simulink model "RTex"  (Simulink 6.0)
settings: Solver=ode3  StartTime=0.0  StopTime=10  FixedStep=0.25  RelTol=1e-3
settings Model: LastModifiedBy=ugur  ExtModeTrigMode=oneshot  ExtModeArmWhenConnect=off
settings ConfigSet: SimulationMode=accelerator
settings DataIOCC: LimitDataPoints=off  SignalLoggingName=sigsOut
settings OptimizationCC: BlockReduction=off  BooleanDataType=off  InlineInvariantSignals=off  LocalBlockOutputs=off
settings DebuggingCC: SolverPrmCheckMsg=none
settings HardwareCC: TargetHWDeviceType=32-bit Generic  ProdEqTarget=off
settings RTWCC: MakeCommand="make_rtw S_FUNCTIONS_LIB=\"..\\rt.lib ..\\winmm.lib\""

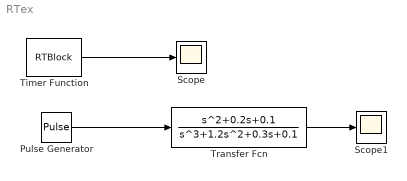
== system RTex ==
  Pulse Generator : DiscretePulseGenerator  PulseType=Time based  Period=1  PulseWidth=50
  Scope : Scope
      settings: YMin=0  YMax=500  SaveName=timing  DataFormat=Array
  Scope1 : Scope
      settings: YMin=0.375  YMax=0.625
  Timer Function : S-Function  FunctionName=RTBlock  Parameters=step,priority,ThPriority  mask(RTBlock){step=250, priority=NORMAL, ThPriority=NORMAL}
      mask prompts: step "Timestep (ms)"; ThPriority "Thread Priority"
      mask help:
      | Real Time Block: Set the characteristics of a real-time simulation. The settings of the simulation are selectable using the block panel. The parameters are:
      |
      | - Timeout: in milliseconds, defines the temporization with which Simulink requires to the Operating System the availability of resources for the execution of the simulation step. The value should be fixed equal to the simulation step of Simulink (the timestep);
      |
      | - Priority Class: defines the class of task priority required, that can be one of the following values:
      | -- IDLE PRIORITY: Low priority, typical of an idle process (priority less than normal)
      | -- NORMAL PRIORITY: Typical priority of a typical windows application;
      | -- HIGH PRIORITY: Typical priority of a relevant application, that needs more resources of a normal application;
      | -- REAL-TIME PRIORITY: Exclusive priority of a unique process that needs all the resources of the operating system.
      |
      | - Thread Priority: defines the class of task priority required, that can be one of the following values:
      | -- IDLE : The thread should run when the main process is inactive.
      | -- LOWEST : The thread runs with a minimal respect of the temporization;
      | -- NORMAL : The thread runs with the same priority of the main process;
      | -- HIGH : The thread runs with the major priority respect to the main process;
      | -- REAL-TIME : The process runs when the simulation thread is in idle state.
      mask StyleString: edit,popup(IDLE|NORMAL|HIGH|REAL-TIME),popup(IDLE|LOWEST|NORMAL|HIGHEST|TIME CRITICAL)
  Transfer Fcn : TransferFcn  Numerator=[1 0.2 0.1]  Denominator=[1 1.2 0.3 0.1]
  wires:
  Timer Function/1 -> Scope/1
  Pulse Generator/1 -> Transfer Fcn/1
  Transfer Fcn/1 -> Scope1/1
